simulink model "arm_sim"  (Simulink 7.7)
settings: Solver=ode45  StartTime=0.0  StopTime=100  RelTol=1e-3
values from neighbouring files (symbols this model uses):
  kd = AP.m*AP.ell^2/3*2*zeta*wn-AP.b    [param.m]
  kp = (AP.tau_max-AP.tau_e)/A_th    [param.m]
undefined symbols (not defined in the file or in its folder): AP, drawArm
settings Model: Creator=beard  LastModifiedBy=beard
settings OptimizationCC: InitFltsAndDblsToZero=on
settings DebuggingCC: StrictBusMsg=Warning

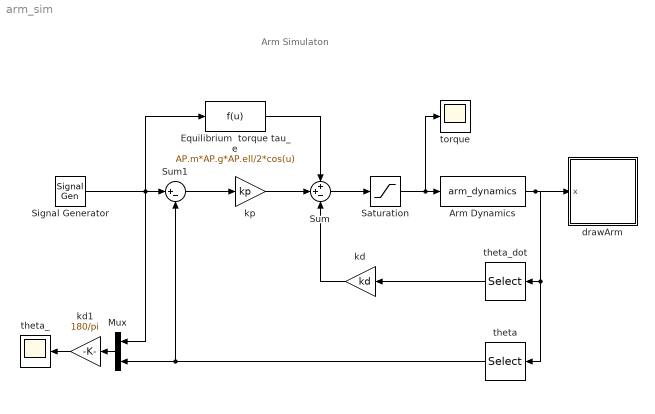
== system arm_sim ==
  note: Arm Simulaton
  Arm Dynamics : S-Function  FunctionName=arm_dynamics  Parameters=AP  EnableBusSupport=off
  Equilibrium  torque tau_e : Fcn  Expr=AP.m*AP.g*AP.ell/2*cos(u)
  Mux : Mux  Inputs=2
  Saturation : Saturate  UpperLimit=1  LowerLimit=-1
  Signal Generator : SignalGenerator  WaveForm=square  Amplitude=25*pi/180  Frequency=.05
  Sum : Sum  Inputs=++-
  Sum1 : Sum  Inputs=|+-
  drawArm : Subsystem
      mask init:
      | % drawing parameters
      | L = 1;
      | w = 0.3;
      mask Display: image(imread('tv.jpg'))
  kd : Gain  Gain=kd
  kd1 : Gain  Gain=180/pi
  kp : Gain  Gain=kp
  theta : Selector  InputPortWidth=2  IndexOptions=Index vector (dialog)  Indices=[1]  OutputSizes=1
  theta_ : Scope
      settings: YMin=-30  YMax=27.5
  theta_dot : Selector  InputPortWidth=2  IndexOptions=Index vector (dialog)  Indices=[2]  OutputSizes=1
  torque : Scope
      settings: YMin=-0.8  YMax=1
  wires:
  Arm Dynamics/1 -> drawArm/1(x), theta/1, theta_dot/1
  Saturation/1 -> Arm Dynamics/1, torque/1
  Sum/1 -> Saturation/1
  Sum1/1 -> kp/1
  Signal Generator/1 -> Sum1/1, Equilibrium  torque tau_e/1, Mux/1
  theta_dot/1 -> kd/1
  theta/1 -> Sum1/2, Mux/2
  kd/1 -> Sum/3
  kp/1 -> Sum/2
  Equilibrium  torque tau_e/1 -> Sum/1
  Mux/1 -> kd1/1
  kd1/1 -> theta_/1

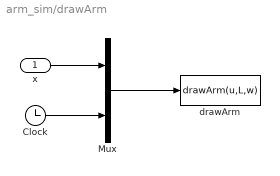
== system arm_sim/drawArm ==
  x : Inport
  Clock : Clock
      settings: Decimation=10
  Mux : Mux  Inputs=2
  drawArm : MATLABFcn  MATLABFcn=drawArm(u,L,w)  OutputDimensions=0  SampleTime=0.1
  wires:
  Mux/1 -> drawArm/1
  x/1 -> Mux/1
  Clock/1 -> Mux/2
